simulink subsystem "weight_extraction_cell"  (R2020b)
settings: Solver=VariableStepAuto  StartTime=0.0  StopTime=10.0  RelTol=1e-3
libraries: hdlsllib x1
settings Model: Creator=jgentile  LastModifiedBy=jgentile

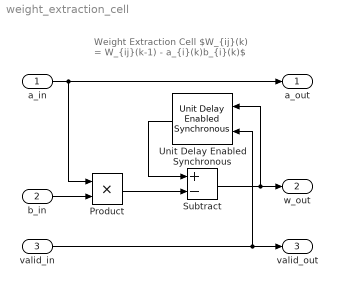
== system weight_extraction_cell ==
  note: Weight Extraction Cell
      | $W_{ij}(k) = W_{ij}(k-1) - a_{i}(k)b_{i}(k)$
  a_in : Inport
  b_in : Inport  Port=2
  valid_in : Inport  Port=3
  Product : Product
  Subtract : Sum  Inputs=+-
  Unit Delay Enabled Synchronous : hdlsllib/Discrete/Unit Delay Enabled Synchronous  InitialCondition=0.0  SampleTime=-1
      settings: SourceProductBaseCode=SL
  a_out : Outport
  w_out : Outport  Port=2
  valid_out : Outport  Port=3
  wires:
  a_in/1 -> Product/1, a_out/1
  b_in/1 -> Product/2
  Product/1 -> Subtract/2
  Subtract/1 -> w_out/1, Unit Delay Enabled Synchronous/1
  Unit Delay Enabled Synchronous/1 -> Subtract/1
  valid_in/1 -> valid_out/1, Unit Delay Enabled Synchronous/2
